simulink model "stepper_model"  (R2018b)
settings: Solver=VariableStepAuto  StartTime=0.0  StopTime=12  FixedStep=0.0001  MaxStep=0.01  RelTol=1e-3  EnableMultiTasking=on
undefined symbols (not defined in the file): jaw_mass, mechanical_hardstop_constraint, position_to_steps, second_arm_mass, st_damping_factor, st_gearbox_damping_factor, st_p_rate, st_pinion_radius, st_rotor_intertia, st_source_voltage_amplitude, third_arm_mass
libraries: fl_lib x38, nesl_utility x16, fl_ps_legacy_lib x8, simulink x1, elec_lib x1, pe_lib x1, sdl_lib x1
settings Model: Creator=The MathWorks, Inc.  LastModifiedBy=Kacper
settings DataIOCC: LimitDataPoints=on
settings OptimizationCC: LifeSpan=inf
settings DebuggingCC: AllowSymbolicDim=off  SFUnexpectedBacktrackingDiag=warning  SFNoUnconditionalDefaultTransitionDiag=warning  SFExecutionAtInitializationDiag=none
settings ModelReferenceCC: PropagateSignalLabelsOutOfModel=off
settings SFSimCC: SimUseLocalCustomCode=off
settings RTWCC: RTWUseLocalCustomCode=off
settings CodeAppCC: StateflowObjectComments=on
settings GRTTargetCC: TargetLangStandard=C89/C90 (ANSI)
settings ConfigComp: CovMetricSettings=dw  CovHtmlReporting=on  CovSaveCumulativeToWorkspaceVar=on  CovSaveSingleToWorkspaceVar=on  CovExternalEMLEnable=off

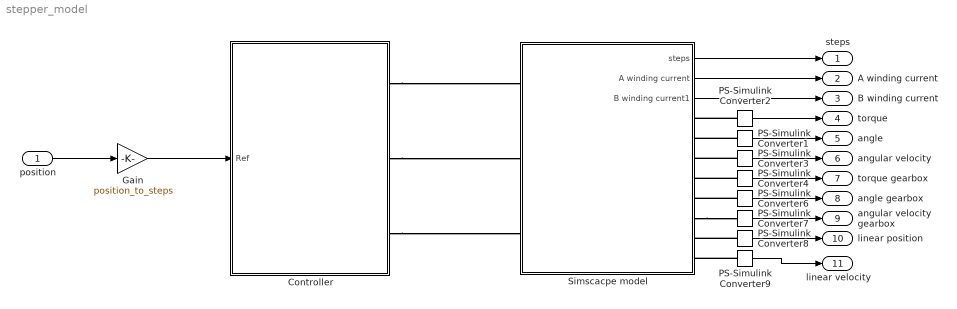
== system stepper_model ==
  position : Inport
  Controller : Subsystem  VariantControlMode=Label  Variant=on  LabelModeActiveChoice=Position
      settings: AttributesFormatString=%<BlockChoice>
  Gain : Gain  Gain=position_to_steps
  PS-Simulink Converter{1..4,6..9} (8 alike) : nesl_utility/PS-Simulink Converter  PhysicalDomain=network_engine_domain  SubClassName=ps_output  LeftPortType=input  RightPortType=output  PseudoPeriodic=off  Frequencies=[]  Unit=1  AffineConversion=off
  Simscacpe model : Subsystem
  steps : Outport
  A winding current : Outport  Port=2
  B winding current : Outport  Port=3
  torque : Outport  Port=4
  angle : Outport  Port=5
  angular velocity : Outport  Port=6
  torque gearbox : Outport  Port=7
  angle gearbox : Outport  Port=8
  angular velocity gearbox : Outport  Port=9
  linear position : Outport  Port=10
  linear velocity : Outport  Port=11
  wires:
  Gain/1 -> Controller/1(Ref)
  Simscacpe model/1("steps ") -> steps/1
  Simscacpe model/2(A winding current) -> A winding current/1
  Simscacpe model/3(B winding current1) -> B winding current/1
  PS-Simulink Converter2/1 -> torque/1
  PS-Simulink Converter1/1 -> angle/1
  PS-Simulink Converter3/1 -> angular velocity/1
  PS-Simulink Converter4/1 -> torque gearbox/1
  PS-Simulink Converter6/1 -> angle gearbox/1
  PS-Simulink Converter7/1 -> angular velocity gearbox/1
  PS-Simulink Converter8/1 -> linear position/1
  PS-Simulink Converter9/1 -> linear velocity/1
  position/1 -> Gain/1
  connections:
  Controller/RConn1 -- Simscacpe model/LConn1
  Controller/RConn2 -- Simscacpe model/LConn2
  Controller/RConn3 -- Simscacpe model/LConn3
  PS-Simulink Converter2/LConn1 -- Simscacpe model/RConn1
  PS-Simulink Converter1/LConn1 -- Simscacpe model/RConn2
  PS-Simulink Converter3/LConn1 -- Simscacpe model/RConn3
  PS-Simulink Converter4/LConn1 -- Simscacpe model/RConn4
  PS-Simulink Converter6/LConn1 -- Simscacpe model/RConn5
  Simscacpe model/RConn6 -- PS-Simulink Converter7/LConn1
  PS-Simulink Converter8/LConn1 -- Simscacpe model/RConn7
  PS-Simulink Converter9/LConn1 -- Simscacpe model/RConn8

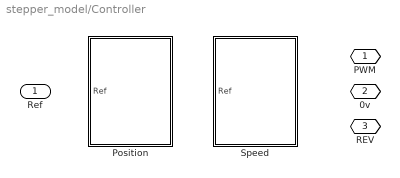
== system stepper_model/Controller ==
  Ref : Inport
  Position : Subsystem  VariantControl=Position
  Speed : Subsystem  VariantControl=Speed
  PWM : PMIOPort  Side=Right
  0v : PMIOPort  Port=2  Side=Right
  REV : PMIOPort  Port=3  Side=Right

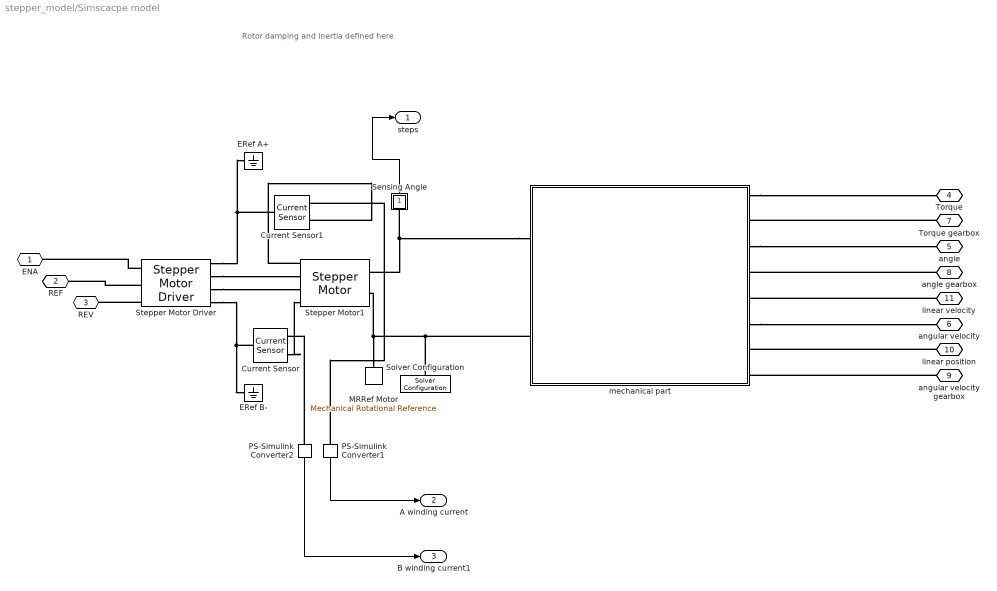
== system stepper_model/Simscacpe model ==
  note: Rotor damping and inertia defined here
  Current Sensor : fl_lib/Electrical/Electrical Sensors/Current Sensor
  Current Sensor1 : fl_lib/Electrical/Electrical Sensors/Current Sensor
  ERef A+ : fl_lib/Electrical/Electrical Elements/Electrical Reference
  ERef B- : fl_lib/Electrical/Electrical Elements/Electrical Reference
  MRRef Motor : fl_lib/Mechanical/Rotational Elements/Mechanical Rotational Reference
  PS-Simulink Converter1 : nesl_utility/PS-Simulink Converter  PhysicalDomain=network_engine_domain  SubClassName=ps_output  LeftPortType=input  RightPortType=output  PseudoPeriodic=off  Frequencies=[]  Unit=1  AffineConversion=off
  PS-Simulink Converter2 : nesl_utility/PS-Simulink Converter  PhysicalDomain=network_engine_domain  SubClassName=ps_output  LeftPortType=input  RightPortType=output  PseudoPeriodic=off  Frequencies=[]  Unit=1  AffineConversion=off
  Sensing Angle : Subsystem
      mask Display: disp('a')
  Solver Configuration : nesl_utility/Solver Configuration  PhysicalDomain=network_engine_domain  SubClassName=solver  LeftPortType=input  RightPortType=generic  Tones=[]  Harmonics=[]  SimulateNoise=off  Profile=off  UseLocalSampling=off  EnableSwitchedLinearOptims=on  FrequencyDomain=off  UseCCode=off  RelTol=0.001  AbsTol=1e-06  MinStep=1e-09  ToWorkspace=off  RevertToSquareIcSolve=off  NumHomotopyIterations=100  PhasorMode=off  PhasorModeNumHarmonics=1  DoDC=off  ResidualTolerance=1e-9  UseLocalSolver=off  LocalSolverChoice=NE_BACKWARD_EULER_ADVANCER  LocalSolverSampleTime=.001  DoFixedCost=off  MaxNonlinIter=3  MaxModeIter=2  LinearAlgebra=auto  EquationFormulation=NE_TIME_EF  DelaysMemoryBudget=1024  AutomaticFiltering=on  FilteringTimeConstant=0.001  PartitionStorageMethod=AS_NEEDED  PartitionMemoryBudget=1024
  Stepper Motor Driver : elec_lib/Actuators & Drivers/Drivers/Stepper Motor Driver  step_or_av=1  step_rate_per_volt=10 Hz/V  Venable=st_source_voltage_amplitude/4 V  Vreverse=st_source_voltage_amplitude/4 V  Vm=st_source_voltage_amplitude V  half_stepping=0
      settings: SourceProductName=Simscape Electronics  SourceProductBaseCode=SN
  Stepper Motor1 : pe_lib/Machines/Stepper Motor and Driver/Stepper Motor  step_or_av=1  w_vec=[0, 1000, 3000] rpm  T_vec=[2, 2, 1] N*m  assert_if_slipping=0  J_total=1e-4 kg*m^2  max_step_rate=10 Hz  Ra=st_winding_resistance Ohm  La=st_winding_inductance H  Km=st_motor_torque_constant N*m/A  Td=st_detent_torque N*m  Rm=st_magnetizing_resistance Ohm  Step=st_full_step_size deg  J=st_rotor_intertia kg*m^2  B=st_damping_factor N*m/(rad/s)  speed0=0 rpm  theta0=0 deg  alpha=[.00393, .00393] 1/K  Tmeas=25 degC  T_vec2=[1.7, 1.7, .85] N*m  Tmeas2=125 degC  half_stepping=0  thermal_masses=[100, 100] J/K  initial_temperatures=[25, 25] degC  rotor_thermal_mass=50 J/K  rotor_initial_temperature=25 degC  Rm_percent_rotor=90
      settings: SourceProductName=Simscape Power Systems  SourceProductBaseCode=PS
  mechanical part : Subsystem
  "ENA " : PMIOPort  Side=Left
  REF : PMIOPort  Port=2  Side=Left
  REV : PMIOPort  Port=3  Side=Left
  Torque : PMIOPort  Port=4  Side=Right
  angle : PMIOPort  Port=5  Side=Right
  angular velocity : PMIOPort  Port=6  Side=Right
  Torque gearbox : PMIOPort  Port=7  Side=Right
  angle gearbox : PMIOPort  Port=8  Side=Right
  angular velocity gearbox : PMIOPort  Port=9  Side=Right
  linear position : PMIOPort  Port=10  Side=Right
  linear velocity : PMIOPort  Port=11  Side=Right
  "steps " : Outport
  A winding current : Outport  Port=2
  B winding current1 : Outport  Port=3
  wires:
  Sensing Angle/1(theta) -> "steps "/1
  PS-Simulink Converter2/1 -> B winding current1/1
  PS-Simulink Converter1/1 -> A winding current/1
  connections:
  Stepper Motor Driver/RConn4 -- Current Sensor/LConn1 -- ERef B-/LConn1
  Stepper Motor Driver/RConn1 -- Current Sensor1/LConn1 -- ERef A+/LConn1
  Solver Configuration/RConn1 -- mechanical part/LConn2 -- Stepper Motor1/RConn2 -- MRRef Motor/LConn1
  Stepper Motor Driver/LConn1 -- "ENA "/RConn1
  mechanical part/LConn1 -- Stepper Motor1/RConn1 -- Sensing Angle/LConn1
  Stepper Motor Driver/LConn3 -- REV/RConn1
  Stepper Motor Driver/LConn2 -- REF/RConn1
  mechanical part/RConn1 -- Torque/RConn1
  Torque gearbox/RConn1 -- mechanical part/RConn2
  mechanical part/RConn3 -- angle/RConn1
  angle gearbox/RConn1 -- mechanical part/RConn4
  linear velocity/RConn1 -- mechanical part/RConn5
  mechanical part/RConn6 -- angular velocity/RConn1
  linear position/RConn1 -- mechanical part/RConn7
  angular velocity gearbox/RConn1 -- mechanical part/RConn8
  Stepper Motor Driver/RConn3 -- Stepper Motor1/LConn3
  Stepper Motor Driver/RConn2 -- Stepper Motor1/LConn2
  Current Sensor/RConn2 -- Stepper Motor1/LConn4
  PS-Simulink Converter2/LConn1 -- Current Sensor/RConn1
  PS-Simulink Converter1/LConn1 -- Current Sensor1/RConn1
  Stepper Motor1/LConn1 -- Current Sensor1/RConn2

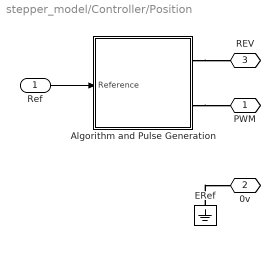
== system stepper_model/Controller/Position ==
  Ref : Inport
  Algorithm and Pulse Generation : Subsystem
  ERef : fl_lib/Electrical/Electrical Elements/Electrical Reference
  PWM : PMIOPort  Side=Right
  0v : PMIOPort  Port=2  Side=Right
  REV : PMIOPort  Port=3  Side=Right
  wires:
  Ref/1 -> Algorithm and Pulse Generation/1(Reference)
  connections:
  ERef/LConn1 -- 0v/RConn1
  Algorithm and Pulse Generation/RConn1 -- REV/RConn1
  Algorithm and Pulse Generation/RConn2 -- PWM/RConn1

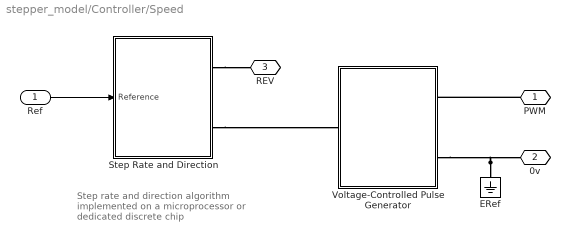
== system stepper_model/Controller/Speed ==
  note: Step rate and direction algorithm implemented on a microprocessor or dedicated discrete chip
  Ref : Inport
  ERef : fl_lib/Electrical/Electrical Elements/Electrical Reference
  Step Rate and Direction : Subsystem
  Voltage-Controlled Pulse Generator : Subsystem
  PWM : PMIOPort  Side=Right
  0v : PMIOPort  Port=2  Side=Right
  REV : PMIOPort  Port=3  Side=Right
  wires:
  Ref/1 -> Step Rate and Direction/1(Reference)
  connections:
  Step Rate and Direction/RConn2 -- Voltage-Controlled Pulse Generator/LConn1
  Step Rate and Direction/RConn1 -- REV/RConn1
  ERef/LConn1 -- 0v/RConn1 -- Voltage-Controlled Pulse Generator/RConn2
  PWM/RConn1 -- Voltage-Controlled Pulse Generator/RConn1

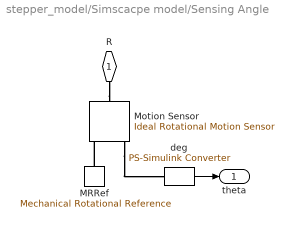
== system stepper_model/Simscacpe model/Sensing Angle ==
  MRRef : fl_lib/Mechanical/Rotational Elements/Mechanical Rotational Reference
  Motion Sensor : fl_lib/Mechanical/Mechanical Sensors/Ideal Rotational Motion Sensor  offset=0 rad
  deg : nesl_utility/PS-Simulink Converter  PhysicalDomain=network_engine_domain  SubClassName=ps_output  LeftPortType=input  RightPortType=output  PseudoPeriodic=off  Frequencies=[]  Unit=deg  AffineConversion=off
  R : PMIOPort  Side=Left
  theta : Outport
  wires:
  deg/1 -> theta/1
  connections:
  R/RConn1 -- Motion Sensor/LConn1
  Motion Sensor/RConn3 -- deg/LConn1
  MRRef/LConn1 -- Motion Sensor/RConn1

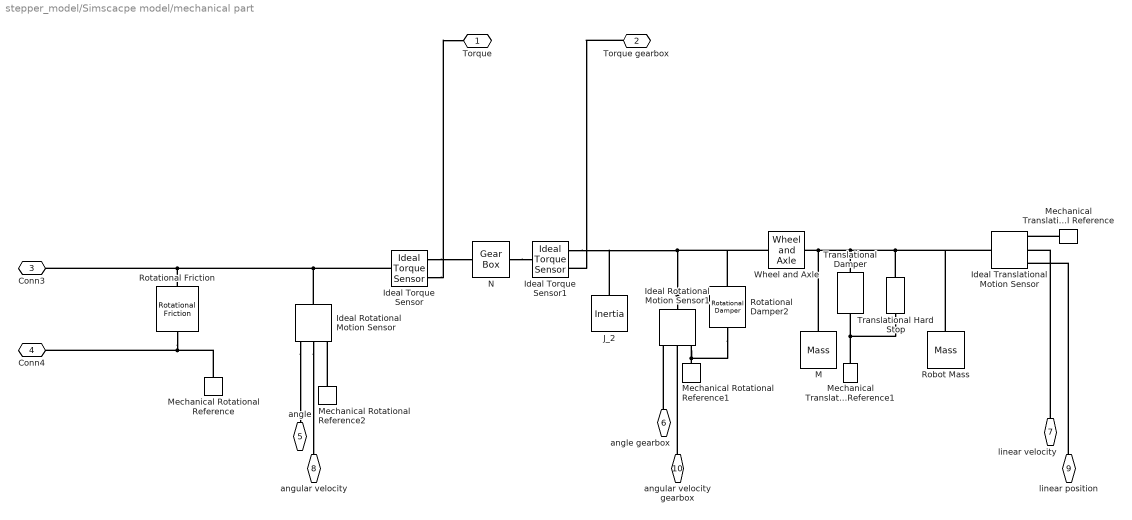
== system stepper_model/Simscacpe model/mechanical part ==
  Ideal Rotational Motion Sensor : fl_lib/Mechanical/Mechanical Sensors/Ideal Rotational Motion Sensor  offset=0 deg
  Ideal Rotational Motion Sensor1 : fl_lib/Mechanical/Mechanical Sensors/Ideal Rotational Motion Sensor  offset=0 rad
  Ideal Torque Sensor : fl_lib/Mechanical/Mechanical Sensors/Ideal Torque Sensor
  Ideal Torque Sensor1 : fl_lib/Mechanical/Mechanical Sensors/Ideal Torque Sensor
  Ideal Translational Motion Sensor : fl_lib/Mechanical/Mechanical Sensors/Ideal Translational Motion Sensor  offset=0 m
  J_2 : fl_lib/Mechanical/Rotational Elements/Inertia  inertia=st_gear_out_inertia kg*m^2  w_specify=off  w_priority=High  w=0 rad/s  w_nominal_specify=off  w_nominal_unit=rad/s  w_nominal_value=1  t_specify=off  t_priority=None  t=1 N*m  t_nominal_specify=off  t_nominal_unit=N*m  t_nominal_value=1
  M : fl_lib/Mechanical/Translational Elements/Mass  mass=st_rack_mass kg  v_specify=off  v_priority=High  v=0 m/s  v_nominal_specify=off  v_nominal_unit=m/s  v_nominal_value=1  f_specify=off  f_priority=None  f=0 N  f_nominal_specify=off  f_nominal_unit=N  f_nominal_value=1
  Mechanical Rotational Reference : fl_lib/Mechanical/Rotational Elements/Mechanical Rotational Reference
  Mechanical Rotational Reference1 : fl_lib/Mechanical/Rotational Elements/Mechanical Rotational Reference
  Mechanical Rotational Reference2 : fl_lib/Mechanical/Rotational Elements/Mechanical Rotational Reference
  Mechanical Translational Reference : fl_lib/Mechanical/Translational Elements/Mechanical Translational Reference
  Mechanical Translational Reference1 : fl_lib/Mechanical/Translational Elements/Mechanical Translational Reference
  N : fl_lib/Mechanical/Mechanisms/Gear Box  ratio=st_gear_ratio  t_in_specify=off  t_in_priority=None  t_in=0 N*m  t_in_nominal_specify=off  t_in_nominal_unit=N*m  t_in_nominal_value=1  t_out_specify=off  t_out_priority=None  t_out=0 N*m  t_out_nominal_specify=off  t_out_nominal_unit=N*m  t_out_nominal_value=1
  Robot Mass : fl_lib/Mechanical/Translational Elements/Mass  mass=second_arm_mass + third_arm_mass + jaw_mass*2 kg  v_specify=off  v_priority=High  v=0 m/s  v_nominal_specify=off  v_nominal_unit=m/s  v_nominal_value=1  f_specify=off  f_priority=None  f=0 N  f_nominal_specify=off  f_nominal_unit=N  f_nominal_value=1
  Rotational Damper2 : fl_lib/Mechanical/Rotational Elements/Rotational Damper  D=st_gearbox_damping_factor N*m/(rad/s)  w_specify=off  w_priority=None  w=0 rad/s  w_nominal_specify=off  w_nominal_unit=rad/s  w_nominal_value=1  t_specify=off  t_priority=None  t=0 N*m  t_nominal_specify=off  t_nominal_unit=N*m  t_nominal_value=1
  Rotational Friction : fl_lib/Mechanical/Rotational Elements/Rotational Friction  brkwy_trq=st_breakaway_friction_torque N*m  brkwy_vel=st_breakaway_friction_velocity rad/s  Col_trq=st_friction_torque N*m  visc_coef=0 N*m/(rad/s)  w_specify=off  w_priority=None  w=0 rad/s  w_nominal_specify=off  w_nominal_unit=rad/s  w_nominal_value=1  t_specify=off  t_priority=None  t=0 N*m  t_nominal_specify=off  t_nominal_unit=N*m  t_nominal_value=1
      settings: SourceProductName=Simscape
  Translational Damper : sdl_lib/Couplings & Drives/Springs & Dampers/Translational Damper  D=0.1 N/(m/s)  enable_faults=0  b_fault=1e6 N/(m/s)  temporal_fault=0  fault_time=5 s  shock_fault=0  acceleration_limit=100 m/s^2  shock_limit=1  report_fault=1
      settings: SourceProductName=Simscape Driveline  SourceProductBaseCode=LD
  Translational Hard Stop : fl_lib/Mechanical/Translational Elements/Translational Hard Stop  upper_bnd=mechanical_hardstop_constraint m  lower_bnd=-mechanical_hardstop_constraint m  stiff_up=1e6 N/m  stiff_low=1e6 N/m  D_up=150 N/(m/s)  D_low=150 N/(m/s)  model=1  transition=0.1 mm  v_specify=off  v_priority=None  v=0 m/s  v_nominal_specify=off  v_nominal_unit=m/s  v_nominal_value=1  f_specify=off  f_priority=None  f=0 N  f_nominal_specify=off  f_nominal_unit=N  f_nominal_value=1  x_specify=off  x_priority=High  x=0 m  x_nominal_specify=off  x_nominal_unit=m  x_nominal_value=1
  Wheel and Axle : fl_lib/Mechanical/Mechanisms/Wheel and Axle  R=st_pinion_radius m  or=1  t_specify=off  t_priority=None  t=0 N*m  t_nominal_specify=off  t_nominal_unit=N*m  t_nominal_value=1  f_specify=off  f_priority=None  f=0 N  f_nominal_specify=off  f_nominal_unit=N  f_nominal_value=1
      settings: SourceProductName=Simscape
  Torque : PMIOPort  Side=Right
  Torque gearbox : PMIOPort  Port=2  Side=Right
  Conn3 : PMIOPort  Port=3  Side=Left
  Conn4 : PMIOPort  Port=4  Side=Left
  angle : PMIOPort  Port=5  Side=Right
  angle gearbox : PMIOPort  Port=6  Side=Right
  linear velocity : PMIOPort  Port=7  Side=Right
  angular velocity : PMIOPort  Port=8  Side=Right
  linear position : PMIOPort  Port=9  Side=Right
  angular velocity gearbox : PMIOPort  Port=10  Side=Right
  connections:
  Torque gearbox/RConn1 -- Ideal Torque Sensor1/RConn2
  Mechanical Rotational Reference1/LConn1 -- Rotational Damper2/RConn1 -- Ideal Rotational Motion Sensor1/RConn1
  Ideal Rotational Motion Sensor1/LConn1 -- Rotational Damper2/LConn1 -- Wheel and Axle/LConn1 -- J_2/LConn1 -- Ideal Torque Sensor1/RConn1
  linear position/RConn1 -- Ideal Translational Motion Sensor/RConn3
  Ideal Rotational Motion Sensor/RConn3 -- angle/RConn1
  Ideal Torque Sensor/LConn1 -- Ideal Rotational Motion Sensor/LConn1 -- Rotational Friction/LConn1 -- Conn3/RConn1
  angle gearbox/RConn1 -- Ideal Rotational Motion Sensor1/RConn3
  Mechanical Translational Reference/LConn1 -- Ideal Translational Motion Sensor/RConn1
  Wheel and Axle/RConn1 -- Translational Hard Stop/LConn1 -- Robot Mass/LConn1 -- Ideal Translational Motion Sensor/LConn1 -- Translational Damper/LConn1 -- M/LConn1
  linear velocity/RConn1 -- Ideal Translational Motion Sensor/RConn2
  Ideal Torque Sensor/RConn1 -- N/LConn1
  Ideal Rotational Motion Sensor/RConn2 -- angular velocity/RConn1
  Ideal Torque Sensor/RConn2 -- Torque/RConn1
  N/RConn1 -- Ideal Torque Sensor1/LConn1
  angular velocity gearbox/RConn1 -- Ideal Rotational Motion Sensor1/RConn2
  Mechanical Rotational Reference2/LConn1 -- Ideal Rotational Motion Sensor/RConn1
  Mechanical Rotational Reference/LConn1 -- Rotational Friction/RConn1 -- Conn4/RConn1
  Mechanical Translational Reference1/LConn1 -- Translational Hard Stop/RConn1 -- Translational Damper/RConn1

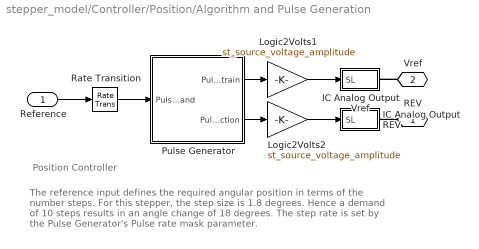
== system stepper_model/Controller/Position/Algorithm and Pulse Generation ==
  note: Position Controller
  note: The reference input defines the required angular position in terms of
      | the number steps. For this stepper, the step size is 1.8 degrees. Hence
      | a demand of 10 steps results in an angle change of 18 degrees.
      | The step rate is set by the Pulse Generator's Pulse rate mask parameter.
  Reference : Inport
  IC Analog Output REV : Subsystem
  IC Analog Output Vref : Subsystem
  Logic2Volts1 : Gain  Gain=st_source_voltage_amplitude
  Logic2Volts2 : Gain  Gain=st_source_voltage_amplitude
  Pulse Generator : Subsystem  mask{f=st_p_rate}
      mask prompts: f "Pulse rate"
  Rate Transition : RateTransition  Deterministic=off
  REV : PMIOPort  Side=Right
  Vref : PMIOPort  Port=2  Side=Right
  wires:
  Rate Transition/1 -> Pulse Generator/1(Pulse  demand)
  Pulse Generator/2(Pulse direction) -> Logic2Volts2/1
  Logic2Volts2/1 -> IC Analog Output REV/1(SL)
  Reference/1 -> Rate Transition/1
  Pulse Generator/1(Pulse train) -> Logic2Volts1/1
  Logic2Volts1/1 -> IC Analog Output Vref/1(SL)
  connections:
  REV/RConn1 -- IC Analog Output REV/RConn1
  Vref/RConn1 -- IC Analog Output Vref/RConn1

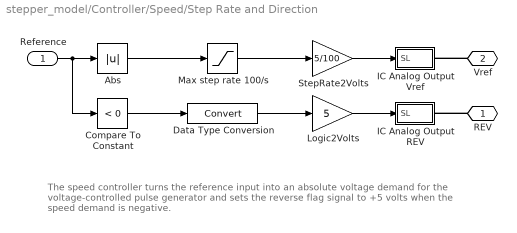
== system stepper_model/Controller/Speed/Step Rate and Direction ==
  note: The speed controller turns the reference input into an absolute voltage demand for the
      | voltage-controlled pulse generator and sets the reverse flag signal to +5 volts when the
      | speed demand is negative.
  Reference : Inport
  Abs : Abs
  Compare To Constant : simulink/Logic and Bit Operations/Compare To Constant  relop=<  const=0  OutDataTypeStr=uint8  ZeroCross=off
  Data Type Conversion : DataTypeConversion
  IC Analog Output REV : Subsystem
  IC Analog Output Vref : Subsystem
  Logic2Volts : Gain  Gain=5
  Max step rate 100/s : Saturate  UpperLimit=100  LowerLimit=0
  StepRate2Volts : Gain  Gain=5/100
  REV : PMIOPort  Side=Right
  Vref : PMIOPort  Port=2  Side=Right
  wires:
  Logic2Volts/1 -> IC Analog Output REV/1(SL)
  Abs/1 -> Max step rate 100/s/1
  Reference/1 -> Abs/1, Compare To Constant/1
  Compare To Constant/1 -> Data Type Conversion/1
  Data Type Conversion/1 -> Logic2Volts/1
  Max step rate 100/s/1 -> StepRate2Volts/1
  StepRate2Volts/1 -> IC Analog Output Vref/1(SL)
  connections:
  Vref/RConn1 -- IC Analog Output Vref/RConn1
  REV/RConn1 -- IC Analog Output REV/RConn1

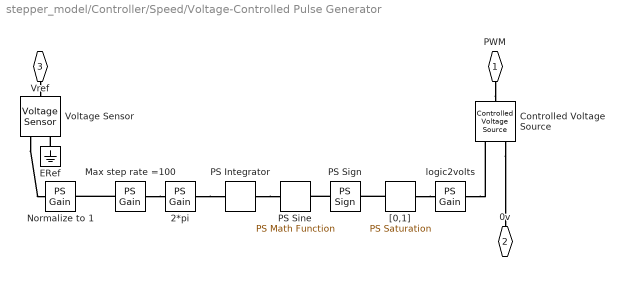
== system stepper_model/Controller/Speed/Voltage-Controlled Pulse Generator ==
  2*pi : fl_ps_legacy_lib/Legacy Physical Signals/Functions/PS Gain  gain=-2*pi
      settings: SourceProductName=Simscape
  Controlled Voltage Source : fl_lib/Electrical/Electrical Sources/Controlled Voltage Source
  ERef : fl_lib/Electrical/Electrical Elements/Electrical Reference
  Max step rate =100 : fl_ps_legacy_lib/Legacy Physical Signals/Functions/PS Gain  gain=100
      settings: SourceProductName=Simscape
  Normalize to 1 : fl_ps_legacy_lib/Legacy Physical Signals/Functions/PS Gain  gain=1/5
      settings: SourceProductName=Simscape
  PS Integrator : fl_ps_legacy_lib/Legacy Physical Signals/Linear Operators/PS Integrator  x0=0
      settings: SourceProductName=Simscape  SourceProductBaseCode=SS
  PS Sign : fl_ps_legacy_lib/Legacy Physical Signals/Nonlinear Operators/PS Sign
      settings: SourceProductName=Simscape  SourceProductBaseCode=SS
  PS Sine : fl_ps_legacy_lib/Legacy Physical Signals/Functions/PS Math Function  fcn_choice=1
      settings: SourceProductName=Simscape  SourceProductBaseCode=SS
  Voltage Sensor : fl_lib/Electrical/Electrical Sensors/Voltage Sensor
  "[0,1]" : fl_ps_legacy_lib/Legacy Physical Signals/Nonlinear Operators/PS Saturation  upper_limit=1  lower_limit=0
      settings: SourceProductName=Simscape  SourceProductBaseCode=SS
  logic2volts : fl_ps_legacy_lib/Legacy Physical Signals/Functions/PS Gain  gain=5
      settings: SourceProductName=Simscape
  PWM : PMIOPort  Side=Right
  0v : PMIOPort  Port=2  Side=Right
  Vref : PMIOPort  Port=3  Side=Left
  connections:
  logic2volts/RConn1 -- Controlled Voltage Source/RConn1
  "[0,1]"/RConn1 -- logic2volts/LConn1
  "[0,1]"/LConn1 -- PS Sign/RConn1
  PS Sign/LConn1 -- PS Sine/RConn1
  PS Integrator/RConn1 -- PS Sine/LConn1
  2*pi/RConn1 -- PS Integrator/LConn1
  Max step rate =100/RConn1 -- 2*pi/LConn1
  Max step rate =100/LConn1 -- Normalize to 1/RConn1
  Voltage Sensor/RConn1 -- Normalize to 1/LConn1
  ERef/LConn1 -- Voltage Sensor/RConn2
  Vref/RConn1 -- Voltage Sensor/LConn1
  Controlled Voltage Source/RConn2 -- 0v/RConn1
  PWM/RConn1 -- Controlled Voltage Source/LConn1

== system stepper_model/Controller/Position/Algorithm and Pulse Generation/IC Analog Output REV ==
  SL : Inport
  Controlled Voltage Source : fl_lib/Electrical/Electrical Sources/Controlled Voltage Source
  ERef : fl_lib/Electrical/Electrical Elements/Electrical Reference
  Simulink-PS Converter : nesl_utility/Simulink-PS Converter  PhysicalDomain=network_engine_domain  SubClassName=ps_input  LeftPortType=input  RightPortType=output  PseudoPeriodic=off  Frequencies=[]  NoiseDistribution=none  NoiseParameters=[]  Unit=V  AffineConversion=off  FilteringAndDerivatives=zero  SimscapeFilterOrder=1  InputFilterTimeConstant=.001  UdotUserProvided=0
  V : PMIOPort  Side=Right
  wires:
  SL/1 -> Simulink-PS Converter/1
  connections:
  Simulink-PS Converter/RConn1 -- Controlled Voltage Source/RConn1
  V/RConn1 -- Controlled Voltage Source/LConn1
  ERef/LConn1 -- Controlled Voltage Source/RConn2

== system stepper_model/Controller/Position/Algorithm and Pulse Generation/IC Analog Output Vref ==
  SL : Inport
  Controlled Voltage Source : fl_lib/Electrical/Electrical Sources/Controlled Voltage Source
  ERef : fl_lib/Electrical/Electrical Elements/Electrical Reference
  Simulink-PS Converter : nesl_utility/Simulink-PS Converter  PhysicalDomain=network_engine_domain  SubClassName=ps_input  LeftPortType=input  RightPortType=output  PseudoPeriodic=off  Frequencies=[]  NoiseDistribution=none  NoiseParameters=[]  Unit=V  AffineConversion=off  FilteringAndDerivatives=zero  SimscapeFilterOrder=1  InputFilterTimeConstant=.001  UdotUserProvided=0
  V : PMIOPort  Side=Right
  wires:
  SL/1 -> Simulink-PS Converter/1
  connections:
  ERef/LConn1 -- Controlled Voltage Source/RConn2
  V/RConn1 -- Controlled Voltage Source/LConn1
  Simulink-PS Converter/RConn1 -- Controlled Voltage Source/RConn1

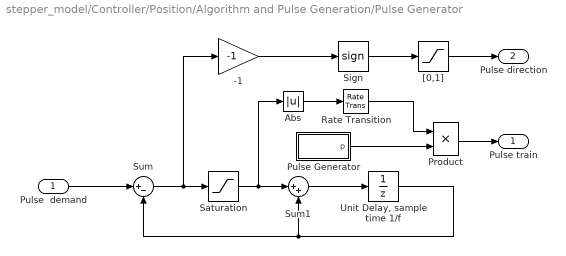
== system stepper_model/Controller/Position/Algorithm and Pulse Generation/Pulse Generator ==
  Pulse  demand : Inport  SampleTime=1/f
  -1 : Gain  Gain=-1
  Abs : Abs
  Product : Product  SaturateOnIntegerOverflow=on  InputSameDT=on  OutDataTypeStr=Inherit: Same as first input
  Pulse Generator : Subsystem
  Rate Transition : RateTransition  Deterministic=off
  Saturation : Saturate  UpperLimit=1  LowerLimit=-1
  Sign : Signum
  Sum : Sum  Inputs=|+-
  Sum1 : Sum  Inputs=|++
  "Unit Delay, sample time 1/f" : UnitDelay  SampleTime=1/f
  "[0,1]" : Saturate  UpperLimit=1  LowerLimit=0
  Pulse train : Outport
  Pulse direction : Outport  Port=2
  wires:
  Rate Transition/1 -> Product/1
  Pulse Generator/1(p) -> Product/2
  Abs/1 -> Rate Transition/1
  Product/1 -> Pulse train/1
  Sign/1 -> "[0,1]"/1
  Sum1/1 -> "Unit Delay, sample time 1/f"/1
  Saturation/1 -> Abs/1, Sum1/1
  Sum/1 -> Saturation/1, -1/1
  Pulse  demand/1 -> Sum/1
  "Unit Delay, sample time 1/f"/1 -> Sum1/2, Sum/2
  -1/1 -> Sign/1
  "[0,1]"/1 -> Pulse direction/1

== system stepper_model/Controller/Speed/Step Rate and Direction/IC Analog Output REV ==
  SL : Inport
  Controlled Voltage Source : fl_lib/Electrical/Electrical Sources/Controlled Voltage Source
  ERef : fl_lib/Electrical/Electrical Elements/Electrical Reference
  Simulink-PS Converter : nesl_utility/Simulink-PS Converter  PhysicalDomain=network_engine_domain  SubClassName=ps_input  LeftPortType=input  RightPortType=output  PseudoPeriodic=off  Frequencies=[]  NoiseDistribution=none  NoiseParameters=[]  Unit=V  AffineConversion=off  FilteringAndDerivatives=zero  SimscapeFilterOrder=1  InputFilterTimeConstant=.001  UdotUserProvided=0
  V : PMIOPort  Side=Right
  wires:
  SL/1 -> Simulink-PS Converter/1
  connections:
  ERef/LConn1 -- Controlled Voltage Source/RConn2
  V/RConn1 -- Controlled Voltage Source/LConn1
  Simulink-PS Converter/RConn1 -- Controlled Voltage Source/RConn1

== system stepper_model/Controller/Speed/Step Rate and Direction/IC Analog Output Vref ==
  SL : Inport
  Controlled Voltage Source : fl_lib/Electrical/Electrical Sources/Controlled Voltage Source
  ERef : fl_lib/Electrical/Electrical Elements/Electrical Reference
  Simulink-PS Converter : nesl_utility/Simulink-PS Converter  PhysicalDomain=network_engine_domain  SubClassName=ps_input  LeftPortType=input  RightPortType=output  PseudoPeriodic=off  Frequencies=[]  NoiseDistribution=none  NoiseParameters=[]  Unit=V  AffineConversion=off  FilteringAndDerivatives=zero  SimscapeFilterOrder=1  InputFilterTimeConstant=.001  UdotUserProvided=0
  V : PMIOPort  Side=Right
  wires:
  SL/1 -> Simulink-PS Converter/1
  connections:
  Simulink-PS Converter/RConn1 -- Controlled Voltage Source/RConn1
  V/RConn1 -- Controlled Voltage Source/LConn1
  ERef/LConn1 -- Controlled Voltage Source/RConn2

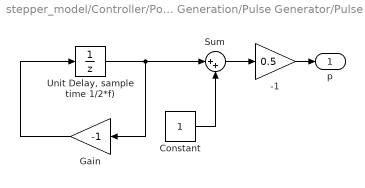
== system stepper_model/Controller/Position/Algorithm and Pulse Generation/Pulse Generator/Pulse Generator ==
  -1 : Gain  Gain=0.5
  Constant : Constant  SampleTime=1/(2*f)
  Gain : Gain  Gain=-1
  Sum : Sum  Inputs=|++
  "Unit Delay, sample time 1/2*f)" : UnitDelay  InitialCondition=-1  SampleTime=1/(2*f)
  p : Outport
  wires:
  -1/1 -> p/1
  Sum/1 -> -1/1
  Constant/1 -> Sum/2
  Gain/1 -> "Unit Delay, sample time 1/2*f)"/1
  "Unit Delay, sample time 1/2*f)"/1 -> Sum/1, Gain/1
